simulink model "Ford_T3T6_ArchCnctnDigrm"  (R2016b)
settings: Solver=FixedStepDiscrete  StartTime=0.0  StopTime=10.0  RelTol=1e-3  EnableMultiTasking=on
libraries: canmsglib x15
(part 5 of 15)

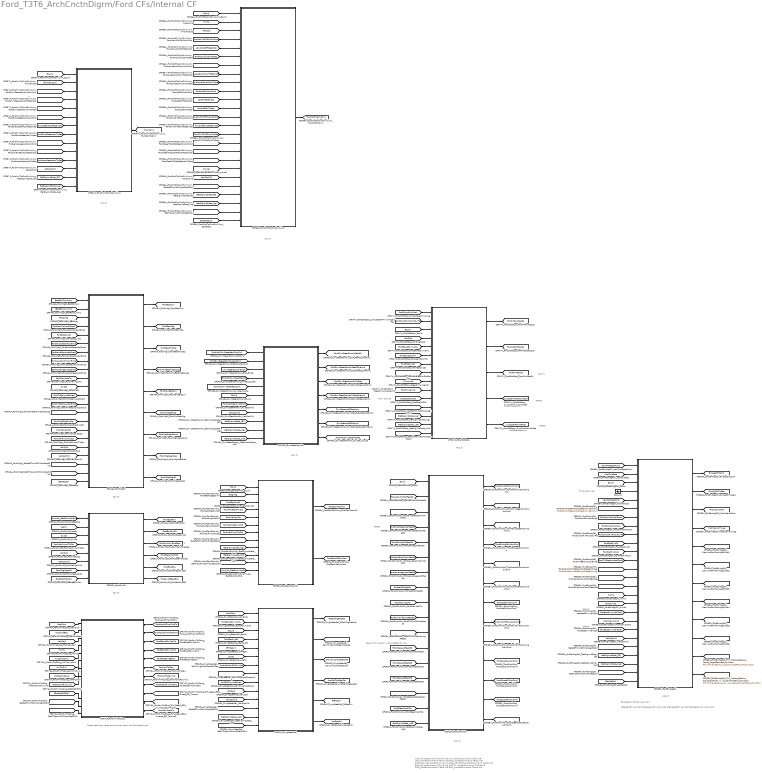
== system Ford_T3T6_ArchCnctnDigrm/Ford CFs/Internal CF ==
  note: CF049
  note: To be removed
  note: A
  note: ??
  note: Takes data from base eps and converts into Ford data type
  note: CAN Tx
  note: SF005
  note: SF005
  note: Spare! Will remain unconnected for now
  note: CF092
  note: LeftLeastDrivenVehicleSpeed
      | kph
      | U-16
      | 1/64
      |
      | RightLeastDrivenVehicleSpeed
      | kph
      | U-16
      | 1/64
  note: EAC_Status
      | Table
      | U-16
      | 1/64
  note: ANC_ArbiterCommand
      | Table
      | U-8
      |
      | LKA_ArbiterCommand
      | Table
      | U-8
      |
      | LDW_ArbiterCommand
      | Table
      | U-8
      |
      | PDC_ArbiterCommand
      | Table
      | U-8
      |
      | PDCLearning_ArbiterCommand
      | Table
      | U-8
      |
      | STDR_ArbiterCommand
      | Table
      | U-8
      |
      | ESA_ArbiterCommand
      | Table
      | U-8
      |
      | LATCTL_ArbiterCommand
      | Table
      | U-8
      |
      | DSR_ArbiterCommand
      | Table
      | U-8
      |
      | EAC_ArbiterCommand
      | Table
      | U-8
  note: ASIL B
  note: ASIL B
  note: ASIL D
  note: ASIL D
  note: ASIL D
  note: ASIL D
  note: ASIL D
  note: StrtStopRateLimit
  note: StrtStopScaleFctr
  note: ASIL D
  note: From DID CF
  note: CF049
  CF046A_FordVltgIf : Subsystem  Tag=1.0.0  Description=This function will inhibit battery voltage diagnostics, define primaryvoltage states and define transitions between battery voltage states
      settings: AttributesFormatString=Version: %<Tag>
  CF047A_FordStrtStop : Subsystem  Tag=1.0.X  Description=Start/Stop is a vehicle event where, to achieve fuel economy,the PCM automatically halts the vehicle engine when the vehicle is stopped and restarts the engine in response to driver commands to resume movement.
      settings: AttributesFormatString=Version: %<Tag>
  CF048A_DrvrSteerRcmdn : Subsystem  Tag=1.0.X  Description=The Driver Steering Recommendation (DSR) function isdesigned to guide the driver to follow/execute a steeringcommand during a split-mu braking or over/understeer condition.This guided steering command is applied in an effort to stabilizethe vehicle and reducing the braking distance in split-mu situations.
      settings: AttributesFormatString=Version: %<Tag>
  CF050A_FordCanDtcInhb : Subsystem  Tag=2.0.X  Description=This function will inhibit requested CAN DTC messagesfor Ford vehicles.This module inhibits CAN DTC messages based on Ford requirements
      settings: AttributesFormatString=Version: %<Tag>
  CF052A_FordSysSt : Subsystem  Tag=1.0.X  Description=Ford System State will handle the internal states and failure modes and output the correct current state to the bus.
      settings: AttributesFormatString=Version: %<Tag>
  CF063A_DrvgSteerSel : Subsystem  Tag=1.0.X  Description=The Driving Steering Select function is a feature which selects different steering modes, safely modifying the steering feel with pre-defined tunings within a given power cycle.
      settings: AttributesFormatString=Version: %<Tag>
  CF065A_FordCmdArbn : Subsystem  Tag=1.0.X  Description=The Ford Arbiter is a function that takes inputs from functions that provide torque overlaysand decides which of those functions may be active and allowed provide a torque overlay
      settings: AttributesFormatString=Version: %<Tag>
  CF066A_FordMotTqCmdOvrlLimr : Subsystem  Tag=1.0.X  Description=The Motor Torque Limiter Function shall sum and limit all output Torque Overlays from Ford features and output them as a value in Motor Nm to be added to the Motor Torque (post-boost curve overlay)
      settings: AttributesFormatString=Version: %<Tag>
  CF067A_FordHwTqCmdOvrlLimr : Subsystem  Tag=1.0.X  Description=The Torque Limiter Function shall sum and limit all inputTorque Overlays from Ford features and output them as avalue in Handwheel Nm to be added to the Handwheel Torque(pre-boost curve overlay)
      settings: AttributesFormatString=Version: %<Tag>
  CF068A_FordExtAgCtrl : Subsystem  Tag=1.0.X  Description=Ford External Angle Control is a function used to process actuationcommands from Ford features into an angle command that can be usedby Nexteer internal functions.
      settings: AttributesFormatString=Version: %<Tag>
  CF076A_FordHwTqCdng : Subsystem  Tag=1.0.X  Description=This function will output various torques in HWNm.It will also calculate an inverse boost curve and outputa percent of available torque for Ford In House Features.
      settings: AttributesFormatString=Version: %<Tag>
  Ground : Ground
  tag scope: DrvrSteerActStPostImc=global, DrvrSteerActStPreImc=global, ExtAgCtrlStsInt=global, ExtAgCtrlTqReq=global, FIH_Read_EPS_Direct_BC_Torque=global, FIH_Read_EPS_Inverse_BC_Torque=global, FIH_Trailer_Backup_Assist_AngleRequest_Function=global, FIH_Trailer_Backup_Assist_External_Angle_ControlStatus_Function=global, FordActvNiblCtrlArbnCmd=global, FordAppldFinalMotTq=global, FordAppldFinalMotTqVld=global, FordBoostCrvAssiTq=global, FordBoostCrvInpTq=global, FordCanDtcInhb=global, FordDrvrSteerRcmdnArbnCmd=global, FordDrvrSteerRcmdnFeatSt=global, FordDrvrSteerRcmdnFeatStPreImc=global, FordDrvrSteerRcmdnTqReq=global, FordDrvrSteerRcmdnTqReqPreImc=global, FordEpsCurr=global, FordEpsEna=global, FordEpsFailr=global, FordEpsLifeCycMod=global, FordEpsSysSt=global, FordEpsVltg=global, FordEvasSteerAssiArbnCmd=global, FordExtAgCtrlArbnCmd=global, FordFeatDircBCTq=global, FordFeatThdSts=global, FordInhbBattVltgDiagc=global, FordInpTqRaw=global, FordInpTqRawVld=global, FordIntPwrReqSt=global, FordIntStrtStopSt=global, FordLaneDprtrWarnArbnCmd=global, FordLaneKeepAssiArbnCmd=global, FordLatCtrlArbnCmd=global, FordMaxAsscTq=global, FordMaxBattCurr=global, FordMinBattVltg=global, FordMotTqCmdOvrl=global, FordPullDriftCmpArbnCmd=global, FordPullDriftCmpLrngArbnCmd=global, FordPwrReqSt=global, FordPwrSplyEnaReq=global, FordReqdFinalMotTq=global, FordSpare1ArbnCmd=global, FordSpare2ArbnCmd=global, FordSpare3ArbnCmd=global, FordSteerDstbcRejctnArbnCmd=global, FordSteerModlSts=global, FordSysStReqEna=global, FordVehDrvrSteerTqReq=global, FordVltgOperRamp=global, FordVltgOperScar=global, FordVltgOperSt=global, HwTqOvrl=global, PosnServoEna=global, PosnServoHwAg=global, RtCalChgReqSts=global, RtReqSrv=global, SelvDrvgModSteerModReq=global, SelvDrvgModSteerSts=global, SemiAutParlParkAgCtrlSts1=global, SemiAutParlParkAgCtrlSts2=global, SemiAutParlParkAgCtrlSts3=global, SemiAutParlParkAgCtrlSts4=global, SemiAutParlParkAgCtrlSts5=global, SemiAutParlParkAgCtrlSts6=global, SysOperMotTqCmdSca=global, SysOperRampRate=global, XcpCalChgReqSts=global, XcpReqSrv=global
  wires:
  [BattRtnCurrAmpr] -> CF046A_FordVltgIf/1(BattRtnCurr)
  [BattRtnCurrImc] -> CF046A_FordVltgIf/2(BattRtnCurrImc)
  [BrdgVltg] -> CF046A_FordVltgIf/3(BattVltg)
  [FordActvParkAssiEnad] -> CF046A_FordVltgIf/4(FordActvParkAssiEnad)
  [FordEpsSysSt] -> CF046A_FordVltgIf/5(FordEpsSysSt)
  [FordEvasSteerAssiEnad] -> CF046A_FordVltgIf/6(FordEvasSteerAssiEnad)
  [FordLaneCentrAssiEnad] -> CF046A_FordVltgIf/7(FordLaneCentrAssiEnad)
  [FordLaneDprtrWarnEnad] -> CF046A_FordVltgIf/8(FordLaneDprtrWarnEnad)
  [FordLaneKeepAssiEnad] -> CF046A_FordVltgIf/9(FordLaneKeepAssiEnad)
  [FordMaxAsscTq] -> CF046A_FordVltgIf/10(FordMaxAsscTq)
  [SysSt] -> CF046A_FordVltgIf/11(FordSysSt)
  [FordTrfcJamAssiEnad] -> CF046A_FordVltgIf/12(FordTrfcJamAssiEnad)
  [FordTrlrBackupAssiEnad] -> CF046A_FordVltgIf/13(FordTrlrBackupAssiEnad)
  [FordVehElecPwrStrtStopSts] -> CF046A_FordVltgIf/14(FordVehElecPwrStrtStopSts)
  [FordVehElecPwrSts] -> CF046A_FordVltgIf/15(FordVehElecPwrSts)
  [FordVehIgnSts] -> CF046A_FordVltgIf/16(FordVehIgnStsQly)
  [FordVehPwrpkTqSts] -> CF046A_FordVltgIf/17(FordVehPwrpkTqSts)
  [VehSpd] -> CF046A_FordVltgIf/18(FordVehSpd)
  [VehSpdVld] -> CF046A_FordVltgIf/19(FordVehSpdVld)
  [GetRefTmr100MicroSec32bit] -> CF046A_FordVltgIf/20(GetRefTmr100MicroSec32bit)
  [GetTiSpan100MicroSec32bit] -> CF046A_FordVltgIf/21(GetTiSpan100MicroSec32bit)
  [SetNtcSts] -> CF046A_FordVltgIf/22(SetNtcSts)
  CF046A_FordVltgIf/1(FordEpsCurr) -> [FordEpsCurr]
  CF046A_FordVltgIf/2(FordEpsVltg) -> [FordEpsVltg]
  CF046A_FordVltgIf/3(FordFeatThdSts) -> [FordFeatThdSts]
  CF046A_FordVltgIf/4(FordInhbBattVltgDiagc) -> [FordInhbBattVltgDiagc]
  CF046A_FordVltgIf/5(FordMaxBattCurr) -> [FordMaxBattCurr]
  CF046A_FordVltgIf/6(FordMinBattVltg) -> [FordMinBattVltg]
  CF046A_FordVltgIf/7(FordVltgOperRamp) -> [FordVltgOperRamp]
  CF046A_FordVltgIf/8(FordVltgOperScar) -> [FordVltgOperScar]
  CF046A_FordVltgIf/9(FordVltgOperSt) -> [FordVltgOperSt]
  [IoHwAb_GetGpioMcuEna] -> CF052A_FordSysSt/1(IoHwAb_GetGpioMcuEna)
  [LoaSt] -> CF052A_FordSysSt/2(LoaSt)
  [SysSt] -> CF052A_FordSysSt/3(SysSt)
  [FordVehPwrpkTqSts] -> CF052A_FordSysSt/4(FordVehPwrpkTqSts)
  [VehSpd] -> CF052A_FordSysSt/5(FordVehSpd)
  [VehSpdVld] -> CF052A_FordSysSt/6(FordVehSpdVld)
  [FordVltgOperSt] -> CF052A_FordSysSt/7(FordVltgOperSt)
  [GetNtcQlfrSts10] -> CF052A_FordSysSt/8(GetNtcQlfrSts)
  CF052A_FordSysSt/1(FordEpsFailr) -> [FordEpsFailr]
  CF052A_FordSysSt/2(FordEpsSysSt) -> [FordEpsSysSt]
  CF052A_FordSysSt/3(FordPwrSplyEnaReq) -> [FordPwrSplyEnaReq]
  CF052A_FordSysSt/4(FordSteerModlSts) -> [FordSteerModlSts]
  [AssiCmd] -> CF076A_FordHwTqCdng/1(AssiCmd)
  [AssiCmdBas] -> CF076A_FordHwTqCdng/2(AssiCmdBas)
  [VehSpd] -> CF076A_FordHwTqCdng/3(FordVehSpd)
  [HwTq] -> CF076A_FordHwTqCdng/4(HwTq)
  [HysCmpCmd] -> CF076A_FordHwTqCdng/5(HwTqHysOvrl)
  [HwTqOvrl] -> CF076A_FordHwTqCdng/6(HwTqOvrl)
  [MotTqCmdSwp] -> CF076A_FordHwTqCdng/7(MotTqCmd)
  [MotTqCmdPwrLimd] -> CF076A_FordHwTqCdng/8(MotTqCmdPwrLimd)
  [GetNtcQlfrSts] -> CF076A_FordHwTqCdng/11(GetNtcQlfrSts)
  [GetRefTmr100MicroSec32bit] -> CF076A_FordHwTqCdng/12(GetRefTmr100MicroSec32bit)
  [GetTiSpan100MicroSec32bit] -> CF076A_FordHwTqCdng/13(GetTiSpan100MicroSec32bit)
  CF076A_FordHwTqCdng/1(FordAppldFinalMotTq) -> [FordAppldFinalMotTq]
  CF076A_FordHwTqCdng/2(FordAppldFinalMotTqVld) -> [FordAppldFinalMotTqVld]
  CF076A_FordHwTqCdng/3(FordBoostCrvAssiTq) -> [FordBoostCrvAssiTq]
  CF076A_FordHwTqCdng/4(FordBoostCrvInpTq) -> [FordBoostCrvInpTq]
  CF076A_FordHwTqCdng/5(FordFeatDircBCTq) -> [FordFeatDircBCTq]
  CF076A_FordHwTqCdng/6(FordInpTqRaw) -> [FordInpTqRaw]
  CF076A_FordHwTqCdng/7(FordInpTqRawVld) -> [FordInpTqRawVld]
  CF076A_FordHwTqCdng/8(FordReqdFinalMotTq) -> [FordReqdFinalMotTq]
  CF076A_FordHwTqCdng/9(FIH_Read_EPS_Direct_BC_Torque) -> [FIH_Read_EPS_Direct_BC_Torque]
  CF076A_FordHwTqCdng/10(FIH_Read_EPS_Inverse_BC_Torque) -> [FIH_Read_EPS_Inverse_BC_Torque]
  [ActvRtIdx] -> CF063A_DrvgSteerSel/1(ActvRtIdx)
  [FordBoostCrvInpTq] -> CF063A_DrvgSteerSel/2(BoostCrvInpTq)
  [EcuId] -> CF063A_DrvgSteerSel/3(EcuId)
  [FordEpsSysSt] -> CF063A_DrvgSteerSel/4(EpsSysSt)
  [FltMtgtn] -> CF063A_DrvgSteerSel/5(FltMtgtn)
  [LoaSt] -> CF063A_DrvgSteerSel/6(LoaSt)
  [FordVehPenSelDrvMod] -> CF063A_DrvgSteerSel/7(SelvDrvgModChassis2Req)
  [FordVehSelDrvModChassisVld] -> CF063A_DrvgSteerSel/8(SelvDrvgModChassisVld)
  [FordSelDrvModEnad] -> CF063A_DrvgSteerSel/9(SelvDrvgModEnad)
  [VehSpd] -> CF063A_DrvgSteerSel/10(VehSpd)
  [VehSpdVld] -> CF063A_DrvgSteerSel/11(VehSpdVld)
  [GetRefTmr100MicroSec32bit] -> CF063A_DrvgSteerSel/12(GetRefTmr100MicroSec32bit)
  [GetSigImcData_u08] -> CF063A_DrvgSteerSel/13(GetSigImcData_u08)
  [GetTiSpan100MicroSec32bit] -> CF063A_DrvgSteerSel/14(GetTiSpan100MicroSec32bit)
  CF063A_DrvgSteerSel/1(RtCalChgReqSts) -> [RtCalChgReqSts]
  CF063A_DrvgSteerSel/2(SelvDrvgModSteerModReq) -> [SelvDrvgModSteerModReq]
  CF063A_DrvgSteerSel/3(SelvDrvgModSteerSts) -> [SelvDrvgModSteerSts]
  CF063A_DrvgSteerSel/4(XcpCalChgReqSts) -> [XcpCalChgReqSts]
  CF063A_DrvgSteerSel/5(RtReqSrv) -> [RtReqSrv]
  CF063A_DrvgSteerSel/6(XcpReqSrv) -> [XcpReqSrv]
  [FordVehDrvrSteerReqCmdVld] -> CF048A_DrvrSteerRcmdn/1(DSRVld)
  [FordDrvrSteerRcmdnArbnCmd] -> CF048A_DrvrSteerRcmdn/2(DSR_ArbiterCmd)
  [DrvrSteerRcmdnEnad] -> CF048A_DrvrSteerRcmdn/3(DSR_Enad)
  [FordVehDrvrSteerReqSts] -> CF048A_DrvrSteerRcmdn/4(DrvSte_D_Stat)
  [FordVehDrvrSteerReqCmd] -> CF048A_DrvrSteerRcmdn/5(DrvSte_Tq_Rq)
  [EcuId] -> CF048A_DrvrSteerRcmdn/6(EcuId)
  [FordVehGearRvsStsVld] -> CF048A_DrvrSteerRcmdn/7(RvsGearVld)
  [VehSpdVld] -> CF048A_DrvrSteerRcmdn/8(VehSpdVld)
  [GetSigImcData_f32] -> CF048A_DrvrSteerRcmdn/9(GetImcSigData_f32)
  [GetSigImcData_logl] -> CF048A_DrvrSteerRcmdn/10(GetImcSigData_logl)
  [GetSigImcData_u08] -> CF048A_DrvrSteerRcmdn/11(GetImcSigData_u08)
  CF048A_DrvrSteerRcmdn/1(DSR_FeatSt_PostImc) -> [FordDrvrSteerRcmdnFeatSt]
  CF048A_DrvrSteerRcmdn/2(DSR_FeatSt_PreImc) -> [FordDrvrSteerRcmdnFeatStPreImc]
  CF048A_DrvrSteerRcmdn/3(DSR_TqReq_PostImc) -> [FordDrvrSteerRcmdnTqReq]
  CF048A_DrvrSteerRcmdn/4(DSR_TqReq_PreImc) -> [FordDrvrSteerRcmdnTqReqPreImc]
  CF048A_DrvrSteerRcmdn/5(DrvSteAct_B_Stat_PostImc) -> [DrvrSteerActStPostImc]
  CF048A_DrvrSteerRcmdn/6(DrvSteAct_B_Stat_PreImc) -> [DrvrSteerActStPreImc]
  CF048A_DrvrSteerRcmdn/7(DrvSte_Tq_Act) -> [FordVehDrvrSteerTqReq]
  [EcuId] -> CF065A_FordCmdArbn/1(EcuId)
  [FordActvNiblCtrlFeatSt] -> CF065A_FordCmdArbn/2(FordActvNiblCtrlFeatSt)
  [FordDrvrSteerRcmdnFeatSt] -> CF065A_FordCmdArbn/3(FordDrvrSteerRcmdnFeatSt)
  [FordEvasSteerAssiFeatSt] -> CF065A_FordCmdArbn/4(FordEvasSteerAssiFeatSt)
  [FordExtAgCtrlFeatSt] -> CF065A_FordCmdArbn/5(FordExtAgCtrlFeatSt)
  [FordLaneDprtrWarnFeatSt] -> CF065A_FordCmdArbn/6(FordLaneDprtrWarnFeatSt)
  [FordLaneKeepAssiFeatSt] -> CF065A_FordCmdArbn/7(FordLaneKeepAssiFeatSt)
  [FordLatCtrlFeatSt] -> CF065A_FordCmdArbn/8(FordLatCtrlFeatSt)
  [FordMaxAsscTq] -> CF065A_FordCmdArbn/9(FordMaxAssiTq)
  [FordPullDriftCmpFeatSt] -> CF065A_FordCmdArbn/10(FordPullDriftCmpFeatSt)
  [FordPullDriftCmpLrngFeatSt] -> CF065A_FordCmdArbn/11(FordPullDriftCmpLrngFeatSt)
  [FordSpare1FeatSt] -> CF065A_FordCmdArbn/12(FordSpare1FeatSt)
  [FordSpare2FeatSt] -> CF065A_FordCmdArbn/13(FordSpare2FeatSt)
  [FordSpare3FeatSt] -> CF065A_FordCmdArbn/14(FordSpare3FeatSt)
  [FordSteerDstbcRejctnFeatSt] -> CF065A_FordCmdArbn/15(FordSteerDstbcRejctnFeatSt)
  [FordSteerModlSts] -> CF065A_FordCmdArbn/16(FordSteerModlSts)
  [GetSigImcData_u08] -> CF065A_FordCmdArbn/17(GetSigImcData_u08)
  CF065A_FordCmdArbn/1(FordActvNiblCtrlArbnCmd) -> [FordActvNiblCtrlArbnCmd]
  CF065A_FordCmdArbn/2(FordDrvrSteerRcmdnArbnCmd) -> [FordDrvrSteerRcmdnArbnCmd]
  CF065A_FordCmdArbn/3(FordEvasSteerAssiArbnCmd) -> [FordEvasSteerAssiArbnCmd]
  CF065A_FordCmdArbn/4(FordExtAgCtrlArbnCmd) -> [FordExtAgCtrlArbnCmd]
  CF065A_FordCmdArbn/5(FordLaneDprtrWarnArbnCmd) -> [FordLaneDprtrWarnArbnCmd]
  CF065A_FordCmdArbn/6(FordLaneKeepAssiArbnCmd) -> [FordLaneKeepAssiArbnCmd]
  CF065A_FordCmdArbn/7(FordLatCtrlArbnCmd) -> [FordLatCtrlArbnCmd]
  CF065A_FordCmdArbn/8(FordPullDriftCmpArbnCmd) -> [FordPullDriftCmpArbnCmd]
  CF065A_FordCmdArbn/9(FordPullDriftCmpLrngArbnCmd) -> [FordPullDriftCmpLrngArbnCmd]
  CF065A_FordCmdArbn/10(FordSpare1ArbnCmd) -> [FordSpare1ArbnCmd]
  CF065A_FordCmdArbn/11(FordSpare2ArbnCmd) -> [FordSpare2ArbnCmd]
  CF065A_FordCmdArbn/12(FordSpare3ArbnCmd) -> [FordSpare3ArbnCmd]
  CF065A_FordCmdArbn/13(FordSteerDstbcRejctnArbnCmd) -> [FordSteerDstbcRejctnArbnCmd]
  [FordCmpdHwPosn] -> CF047A_FordStrtStop/1(CmpdSteerPinionAg)
  [FordCmpdHwPosnQlyFac] -> CF047A_FordStrtStop/2(CmpdSteerPinionAgQlyFac)
  [EcuId] -> CF047A_FordStrtStop/3(EcuId)
  [VehSpd] -> CF047A_FordStrtStop/4(FildVehSpd)
  [FordBoostCrvInpTq] -> CF047A_FordStrtStop/5(FordBoostCrvInpTq)
  [FordCanDtcInhb] -> CF047A_FordStrtStop/6(FordCanDtcInhb)
  [FordEpsSysSt] -> CF047A_FordStrtStop/7(FordEpsSysSt)
  [FordVehElecPwrStrtStopSts] -> CF047A_FordStrtStop/8(FordVehElecPwrStrtStopSts)
  [PinionVel] -> CF047A_FordStrtStop/9(SteerPinionAgVel)
  [FordHwVelVld] -> CF047A_FordStrtStop/10(SteerPinionAgVelVld)
  [StrtStopEnadSt] -> CF047A_FordStrtStop/11(StrtStopDIDSt)
  [GetRefTmr100MicroSec32bit] -> CF047A_FordStrtStop/12(GetRefTmr100MicroSec32bit)
  [GetSigImcData_logl] -> CF047A_FordStrtStop/13(GetSigImcData_logl)
  [GetSigImcData_u08] -> CF047A_FordStrtStop/14(GetSigImcData_u08)
  [GetTiSpan100MicroSec32bit] -> CF047A_FordStrtStop/15(GetTiSpan100MicroSec32bit)
  CF047A_FordStrtStop/1(FordIntPwrReqSt) -> [FordIntPwrReqSt]
  CF047A_FordStrtStop/2(FordIntStrtStopSt) -> [FordIntStrtStopSt]
  CF047A_FordStrtStop/3(FordPwrReqSt) -> [FordPwrReqSt]
  CF047A_FordStrtStop/4(SysOperMotTqCmdSca) -> [SysOperMotTqCmdSca]
  CF047A_FordStrtStop/5(SysOperRampRate) -> [SysOperRampRate]
  [EcuId] -> CF066A_FordMotTqCmdOvrlLimr/1(EcuId)
  [HwTq] -> CF066A_FordMotTqCmdOvrlLimr/2(FildHwTq)
  [VehSpd] -> CF066A_FordMotTqCmdOvrlLimr/3(FildVehSpd)
  [FordActvNiblCtrlArbnCmd] -> CF066A_FordMotTqCmdOvrlLimr/4(FordActvNiblCtrlArbnCmd)
  [ActvNiblCtrlFctCallSts] -> CF066A_FordMotTqCmdOvrlLimr/5(FordActvNiblCtrlFctCallSts)
  [FordActvNiblCtrlTqReq] -> CF066A_FordMotTqCmdOvrlLimr/6(FordActvNiblCtrlTqReq)
  [FordLaneDprtrWarnArbnCmd] -> CF066A_FordMotTqCmdOvrlLimr/7(FordLaneDprtrWarnArbnCmd)
  [LaneDprtrWarnFctCallSts] -> CF066A_FordMotTqCmdOvrlLimr/8(FordLaneDprtrWarnFctCallSts)
  [FordLaneDprtrWarnTqReq] -> CF066A_FordMotTqCmdOvrlLimr/9(FordLaneDprtrWarnTqReq)
  [FordLatCtrlArbnCmd] -> CF066A_FordMotTqCmdOvrlLimr/10(FordLatCtrlArbnCmd)
  [LatCtrlFctCallSts] -> CF066A_FordMotTqCmdOvrlLimr/11(FordLatCtrlFctCallSts)
  [FordLatCtrlTqReq] -> CF066A_FordMotTqCmdOvrlLimr/12(FordLatCtrlTqReq)
  [FordPullDriftCmpArbnCmd] -> CF066A_FordMotTqCmdOvrlLimr/13(FordPullDriftCmpArbnCmd)
  [PullDriftCmpFctCallSts] -> CF066A_FordMotTqCmdOvrlLimr/14(FordPullDriftCmpFctCallSts)
  [FordPullDriftCmpTqReq] -> CF066A_FordMotTqCmdOvrlLimr/15(FordPullDriftCmpTqReq)
  [FordSteerDstbcRejctnArbnCmd] -> CF066A_FordMotTqCmdOvrlLimr/16(FordSteerTqDstbcRejctnArbnCmd)
  [SteerTqDstbcRejctnFctCallSts] -> CF066A_FordMotTqCmdOvrlLimr/17(FordSteerTqDstbcRejctnFctCallSts)
  [FordSteerTqDstbcRejctnTqReq] -> CF066A_FordMotTqCmdOvrlLimr/18(FordSteerTqDstbcRejctnTqReq)
  [HwVel] -> CF066A_FordMotTqCmdOvrlLimr/19(HwVel)
  [VehSpdVld] -> CF066A_FordMotTqCmdOvrlLimr/20(VehSpdVld)
  [GetRefTmr100MicroSec32bit] -> CF066A_FordMotTqCmdOvrlLimr/21(GetRefTmr100MicroSec32bit)
  [GetSigImcData_f32] -> CF066A_FordMotTqCmdOvrlLimr/22(GetSigImcData_f32)
  [GetSigImcData_logl] -> CF066A_FordMotTqCmdOvrlLimr/23(GetSigImcData_logl)
  [GetTiSpan100MicroSec32bit] -> CF066A_FordMotTqCmdOvrlLimr/24(GetTiSpan100MicroSec32bit)
  [SetNtcSts10] -> CF066A_FordMotTqCmdOvrlLimr/25(SetNtcSts)
  CF066A_FordMotTqCmdOvrlLimr/1(FordMotTqOvrl) -> [FordMotTqCmdOvrl]
  [EcuId] -> CF067A_FordHwTqCmdOvrlLimr/1(EcuId)
  [FildVehSpd] -> CF067A_FordHwTqCmdOvrlLimr/2(FildVehSpd)
  [FordDrvrSteerRcmdnArbnCmd] -> CF067A_FordHwTqCmdOvrlLimr/3(FordDrvrSteerRcmdnArbnCmd)
  [FordDrvrSteerRcmdnFctCallSts] -> CF067A_FordHwTqCmdOvrlLimr/4(FordDrvrSteerRcmdnFctCallSts)
  [FordDrvrSteerRcmdnTqReq] -> CF067A_FordHwTqCmdOvrlLimr/5(FordDrvrSteerRcmdnTqReq)
  [FordEvasSteerAssiArbnCmd] -> CF067A_FordHwTqCmdOvrlLimr/6(FordEvasSteerAssiArbnCmd)
  [EvasSteerAssiFctCallSts] -> CF067A_FordHwTqCmdOvrlLimr/7(FordEvasSteerAssiFctCallSts)
  [FordEvasSteerAssiTqReq] -> CF067A_FordHwTqCmdOvrlLimr/8(FordEvasSteerAssiTqReq)
  [FordLaneKeepAssiArbnCmd] -> CF067A_FordHwTqCmdOvrlLimr/9(FordLaneKeepAssiArbnCmd)
  [FordLaneKeepAssiFctCallSts] -> CF067A_FordHwTqCmdOvrlLimr/10(FordLaneKeepAssiFctCallSts)
  [FordLaneKeepAssiTqReq] -> CF067A_FordHwTqCmdOvrlLimr/11(FordLaneKeepAssiTqReq)
  [VehSpdVld] -> CF067A_FordHwTqCmdOvrlLimr/12(VehSpdVld)
  [GetSigImcData_f32] -> CF067A_FordHwTqCmdOvrlLimr/13(GetSigImcData_f32)
  [GetSigImcData_logl] -> CF067A_FordHwTqCmdOvrlLimr/14(GetSigImcData_logl)
  CF067A_FordHwTqCmdOvrlLimr/1(FordColTqOvrl) -> [HwTqOvrl]
  [EcuId] -> CF050A_FordCanDtcInhb/1(EcuId)
  [BrdgVltg] -> CF050A_FordCanDtcInhb/2(FordBattVltgEstimn)
  [FordEpsSysSt] -> CF050A_FordCanDtcInhb/3(FordEpsSysSt)
  [FordVehElecPwrSts] -> CF050A_FordCanDtcInhb/4(FordVehElecPwrSts)
  [FordVehIgnSts] -> CF050A_FordCanDtcInhb/5(FordVehIgnStsQly)
  [FordVehLifeCycMod] -> CF050A_FordCanDtcInhb/6(FordVehLifeCycModQly)
  [FordVehPwrpkTqSts] -> CF050A_FordCanDtcInhb/7(FordVehPwrpkTqSts)
  [GetRefTmr100MicroSec32bit] -> CF050A_FordCanDtcInhb/8(GetRefTmr100MicroSec32bit)
  [GetSigImcData_logl] -> CF050A_FordCanDtcInhb/9(GetSigImcData_logl)
  [GetSigImcData_u08] -> CF050A_FordCanDtcInhb/10(GetSigImcData_u08)
  [GetTiSpan100MicroSec32bit] -> CF050A_FordCanDtcInhb/11(GetTiSpan100MicroSec32bit)
  [IoHwAb_GetGpioMcuEna] -> CF050A_FordCanDtcInhb/12(IoHwAb_GetGpioMcuEna)
  CF050A_FordCanDtcInhb/1(FordCanDtcInhb) -> [FordCanDtcInhb]
  CF050A_FordCanDtcInhb/2(FordEpsLifeCycMod) -> [FordEpsLifeCycMod]
  CF076A_FordHwTqCdng/11(FordMaxAsscTq) -> [FordMaxAsscTq]
  CF052A_FordSysSt/5(FordEpsEna) -> [FordEpsEna]
  CF052A_FordSysSt/6(FordSysStReqEna) -> [FordSysStReqEna]
  [ActvFrntSteerPrsnt] -> CF068A_FordExtAgCtrl/1(ActvFrntSteerPrsnt)
  [AssiCmdBas] -> CF068A_FordExtAgCtrl/2(AssiCmdBas)
  [EcuId] -> CF068A_FordExtAgCtrl/3(EcuId)
  Ground/1 -> CF068A_FordExtAgCtrl/4(ExtAgCtrlDiagcFlg)
  [VehSpdSigCdnd] -> CF068A_FordExtAgCtrl/5(FildVehSpd)
  [FordActvFrntSteerModlSteerWhlAgVldInt] -> CF068A_FordExtAgCtrl/6(FordActvFrntSteerModlSteerWhlAgVldInt)
  [FordActvParkAssiEnad] -> CF068A_FordExtAgCtrl/7(FordActvParkAssiEnad)
  [FordCmpdHwPosn] -> CF068A_FordExtAgCtrl/8(FordCmpdHwPosn)
  [FordCmpdHwPosnQlyFac] -> CF068A_FordExtAgCtrl/9(FordCmpdHwPosnQlyFac)
  [FordEpsSysSt] -> CF068A_FordExtAgCtrl/10(FordEpsSysSt)
  [FordRelHwPosn] -> CF068A_FordExtAgCtrl/11(FordRelHwPosn)
  [FordTrlrBackupAssiEnad] -> CF068A_FordExtAgCtrl/12(FordTrlrBackupAssiEnad)
  [FordVehActvFrntSteerModlSteerWhlAg] -> CF068A_FordExtAgCtrl/13(FordVehActvFrntSteerModlSteerWhlAg)
  [FordVehParkAidModlReqdAgPassd] -> CF068A_FordExtAgCtrl/14(FordVehParkAidModlReqdAg)
  [FordVehParkAidModlReqdStsPassd] -> CF068A_FordExtAgCtrl/15(FordVehParkAidModlReqdSts)
  [HwTq] -> CF068A_FordExtAgCtrl/16(HwTq)
  [FordHwVel] -> CF068A_FordExtAgCtrl/17(HwVel)
  [LeLeastDrvnVehSpd] -> CF068A_FordExtAgCtrl/18(LeLeastDrvnVehSpd)
  [PosnServoCmd] -> CF068A_FordExtAgCtrl/19(PosnServoCmd)
  [RiLeastDrvnVehSpd] -> CF068A_FordExtAgCtrl/20(RiLeastDrvnVehSpd)
  [VehSpdVld] -> CF068A_FordExtAgCtrl/21(VehSpdVld)
  [GetRefTmr100MicroSec32bit] -> CF068A_FordExtAgCtrl/22(GetRefTmr100MicroSec32bit)
  [GetSigImcData_f32] -> CF068A_FordExtAgCtrl/23(GetSigImcData_f32)
  [GetSigImcData_logl] -> CF068A_FordExtAgCtrl/24(GetSigImcData_logl)
  [GetTiSpan100MicroSec32bit] -> CF068A_FordExtAgCtrl/25(GetTiSpan100MicroSec32bit)
  [SetNtcSts] -> CF068A_FordExtAgCtrl/26(SetNtcSts)
  CF068A_FordExtAgCtrl/1(ExtAgCtrlStsInt) -> [ExtAgCtrlStsInt]
  CF068A_FordExtAgCtrl/2(ExtAgCtrlTqReq) -> [ExtAgCtrlTqReq]
  CF068A_FordExtAgCtrl/3(PosnServoEna) -> [PosnServoEna]
  CF068A_FordExtAgCtrl/4(PosnServoHwAg) -> [PosnServoHwAg]
  CF068A_FordExtAgCtrl/5(SemiAutParlParkAgCtrlSts1) -> [SemiAutParlParkAgCtrlSts1]
  CF068A_FordExtAgCtrl/6(SemiAutParlParkAgCtrlSts2) -> [SemiAutParlParkAgCtrlSts2]
  CF068A_FordExtAgCtrl/7(SemiAutParlParkAgCtrlSts3) -> [SemiAutParlParkAgCtrlSts3]
  CF068A_FordExtAgCtrl/8(SemiAutParlParkAgCtrlSts4) -> [SemiAutParlParkAgCtrlSts4]
  CF068A_FordExtAgCtrl/9(SemiAutParlParkAgCtrlSts5) -> [SemiAutParlParkAgCtrlSts5]
  CF068A_FordExtAgCtrl/10(SemiAutParlParkAgCtrlSts6) -> [SemiAutParlParkAgCtrlSts6]
  CF068A_FordExtAgCtrl/11(FIH_Trailer_Backup_Assist_AngleRequest_Function) -> [FIH_Trailer_Backup_Assist_AngleRequest_Function]
  CF068A_FordExtAgCtrl/12(FIH_Trailer_Backup_Assist_External_Angle_ControlStatus_Function) -> [FIH_Trailer_Backup_Assist_External_Angle_ControlStatus_Function]

== system Ford_T3T6_ArchCnctnDigrm/Generate Motor Voltage/CM770A_GtmCfgAndUse ==
  MotCurrEolCalSt : Inport
  SysSt : Inport  Port=2
  MotCtrlMotCurrEolCalSt : Inport  Port=3
  MotCtrlPhaOnTiA : Inport  Port=4
  MotCtrlPhaOnTiB : Inport  Port=5
  MotCtrlPhaOnTiC : Inport  Port=6
  MotCtrlPwmPerd : Inport  Port=7
  IoHwAb_SetFctGpioPhaALowrCmd : Inport  Port=8
  IoHwAb_SetFctGpioPhaAUpprCmd : Inport  Port=9
  IoHwAb_SetFctGpioPhaBLowrCmd : Inport  Port=10
  IoHwAb_SetFctGpioPhaBUpprCmd : Inport  Port=11
  IoHwAb_SetFctGpioPhaCLowrCmd : Inport  Port=12
  IoHwAb_SetFctGpioPhaCUpprCmd : Inport  Port=13
  IoHwAb_SetFctPeriphPhaALowrCmd : Inport  Port=14
  IoHwAb_SetFctPeriphPhaAUpprCmd : Inport  Port=15
  IoHwAb_SetFctPeriphPhaBLowrCmd : Inport  Port=16
  IoHwAb_SetFctPeriphPhaBUpprCmd : Inport  Port=17
  IoHwAb_SetFctPeriphPhaCLowrCmd : Inport  Port=18
  IoHwAb_SetFctPeriphPhaCUpprCmd : Inport  Port=19
  IoHwAb_SetGpioPhaALowrCmd : Inport  Port=20
  IoHwAb_SetGpioPhaAUpprCmd : Inport  Port=21
  IoHwAb_SetGpioPhaBLowrCmd : Inport  Port=22
  IoHwAb_SetGpioPhaBUpprCmd : Inport  Port=23
  IoHwAb_SetGpioPhaCLowrCmd : Inport  Port=24
  IoHwAb_SetGpioPhaCUpprCmd : Inport  Port=25
  PhaOnTiMeasdA : Outport
  PhaOnTiMeasdB : Outport  Port=2
  PhaOnTiMeasdC : Outport  Port=3
  GtmGetSent0Data : Outport  Port=4
  GtmGetSent1Data : Outport  Port=5

== system Ford_T3T6_ArchCnctnDigrm/Generate Motor Voltage/ES300A_SinVltgGenn ==
  MotElecMeclPolarity : Inport
  MotCtrlIvtrFetFltPha : Inport  Port=2
  MotCtrlIvtrFetFltTyp : Inport  Port=3
  MotCtrlMfgEnaSt : Inport  Port=4
  MotCtrlMotAgElec : Inport  Port=5
  MotCtrlMotModlnIdx : Inport  Port=6
  MotCtrlMotPhaAdv : Inport  Port=7
  MotCtrlSwCalEna : Inport  Port=8
  MotCtrlSwCalModlnIdx : Inport  Port=9
  MotCtrlSwCalPosnIdx : Inport  Port=10
  MotCtrlVehSpd : Inport  Port=11
  MotCtrlCmuOffs : Outport
  MotCtrlPhaOnTiA : Outport  Port=2
  MotCtrlPhaOnTiB : Outport  Port=3
  MotCtrlPhaOnTiC : Outport  Port=4
  MotCtrlPhaOnTiSumA : Outport  Port=5
  MotCtrlPhaOnTiSumB : Outport  Port=6
  MotCtrlPhaOnTiSumC : Outport  Port=7
  MotCtrlPwmPerd : Outport  Port=8

== system Ford_T3T6_ArchCnctnDigrm/Generate Steering Command/DF002A_Swp ==
  HwTq : Inport
  MotTqCmd : Inport  Port=2
  VehSpd : Inport  Port=3
  VehSpdVld : Inport  Port=4
  GetRefTmr100MicroSec32bit : Inport  Port=5
  GetTiSpan100MicroSec32bit : Inport  Port=6
  HwTqSwp : Outport
  MotTqCmdSwp : Outport  Port=2

== system Ford_T3T6_ArchCnctnDigrm/Generate Steering Command/Openloop Steering Command ==
  HwTqSwp : Inport
  GenerateSteeringCommand : Subsystem
  System Protection : Subsystem
  MotTqCmd : Outport
  wires:
  HwTqSwp/1 -> GenerateSteeringCommand/1(HwTqSwp)
  GenerateSteeringCommand/1(MotTqCmd) -> MotTqCmd/1
  GenerateSteeringCommand/2(MotTqCmdLimdPreStall) -> System Protection/1(MotTqCmdLimdPreStall)
  System Protection/1(EotAssiSca) -> GenerateSteeringCommand/2(EotAssiSca)
  System Protection/2(EotActvCmd) -> GenerateSteeringCommand/3(EotActvCmd)
  System Protection/3(EotDampgCmd) -> GenerateSteeringCommand/4(EotDampgCmd)
  System Protection/4(EotMotTqLim) -> GenerateSteeringCommand/5(EotMotTqLim)
  System Protection/5(StallMotTqLim) -> GenerateSteeringCommand/6(StallMotTqLim)
  System Protection/6(ThermMotTqLim) -> GenerateSteeringCommand/7(ThermMotTqLim)
  System Protection/7(VehSpdMotTqLim) -> GenerateSteeringCommand/8(VehSpdMotTqLim)

== system Ford_T3T6_ArchCnctnDigrm/Imc Com and Arbn/AR350A_ImcArbn ==
  SetNtcSts : Inport
  GetSigImcDataExtdSts_f32 : Outport
  GetSigImcDataExtdSts_logl : Outport  Port=2
  GetSigImcDataExtdSts_s08 : Outport  Port=3
  GetSigImcDataExtdSts_s16 : Outport  Port=4
  GetSigImcDataExtdSts_s32 : Outport  Port=5
  GetSigImcDataExtdSts_u08 : Outport  Port=6
  GetSigImcDataExtdSts_u16 : Outport  Port=7
  GetSigImcDataExtdSts_u32 : Outport  Port=8
  GetSigImcData_f32 : Outport  Port=9
  GetSigImcData_logl : Outport  Port=10
  GetSigImcData_s08 : Outport  Port=11
  GetSigImcData_s16 : Outport  Port=12
  GetSigImcData_s32 : Outport  Port=13
  GetSigImcData_u08 : Outport  Port=14
  GetSigImcData_u16 : Outport  Port=15
  GetSigImcData_u32 : Outport  Port=16
  GetTxRateGroup : Outport  Port=17
  GetTxSigGroup : Outport  Port=18
  SetRxSigGroup : Outport  Port=19

== system Ford_T3T6_ArchCnctnDigrm/Imc Com and Arbn/CM760A_Uart0CfgAndUse ==
  GetTxRateGroup : Inport
  SetRxSigGroup : Inport  Port=2

== system Ford_T3T6_ArchCnctnDigrm/Imc Com and Arbn/CM765A_Uart1CfgAndUse ==
  GetTxRateGroup : Inport
  SetRxSigGroup : Inport  Port=2

== system Ford_T3T6_ArchCnctnDigrm/Imc Com and Arbn/ES011A_DualEcuIdn ==
  EcuComTiOut : Inport
  GetSigImcData_u08 : Inport  Port=2
  IoHwAb_GetGpioEcuIdnPin1 : Inport  Port=3
  IoHwAb_GetGpioEcuIdnPin2 : Inport  Port=4
  SetNtcSts : Inport  Port=5
  EcuId : Outport  OutMin=0  OutMax=4  OutDataTypeStr=uint8

== system Ford_T3T6_ArchCnctnDigrm/Imc Com and Arbn/SF062B_DualCtrlrOutpMgr ==
  ImcSysSt : Inport
  ImcSysStVld : Inport  Port=2
  MotAndThermProtnLoaMod : Inport  Port=3
  SysSt : Inport  Port=4
  VehSpd : Inport  Port=5
  GetRefTmr100MicroSec32bit : Inport  Port=6
  GetSigImcData_logl : Inport  Port=7
  GetTiSpan100MicroSec32bit : Inport  Port=8
  DualEcuFltMtgtnEna : Outport
  DualEcuFltMtgtnSca : Outport  Port=2
  DualEcuMotCtrlMtgtnEna : Outport  Port=3

== system Ford_T3T6_ArchCnctnDigrm/Imc Com and Arbn/SF063A_ImcSigArbn ==
  EcuIdn : Inport
  HwAg : Inport  Port=2
  HwTq : Inport  Port=3
  MotVelCrf : Inport  Port=4
  PosnServoHwAg : Inport  Port=5
  PosnServoIntgtrSt : Inport  Port=6
  PosnTrakgIntgtrSt1 : Inport  Port=7
  PosnTrakgIntgtrSt2 : Inport  Port=8
  PullCmpLongTermIntgtrSt : Inport  Port=9
  PullCmpShoTermIntgtrSt : Inport  Port=10
  VehSpd : Inport  Port=11
  GetRefTmr100MicroSec32bit : Inport  Port=12
  GetSigImcData_f32 : Inport  Port=13
  GetSigImcData_logl : Inport  Port=14
  GetSigImcData_u08 : Inport  Port=15
  GetTiSpan100MicroSec32bit : Inport  Port=16
  SetNtcSts : Inport  Port=17
  HwAgImcCorrd : Outport
  HwTqImcCorrd : Outport  Port=2
  ImcSysSt : Outport  Port=3
  ImcSysStVld : Outport  Port=4
  MotVelCrfImcCorrd : Outport  Port=5
  PosnServoHwAgImcCorrd : Outport  Port=6
  PosnServoIntgtrOffs : Outport  Port=7
  PosnTrakgArbnFltMtgtnEna : Outport  Port=8
  PosnTrakgIntgtrSt1Offs : Outport  Port=9
  PosnTrakgIntgtrSt2Offs : Outport  Port=10
  PullCmpLongTermIntgtrStOffs : Outport  Port=11
  PullCmpShoTermIntgtrStOffs : Outport  Port=12
  VehSpdImcCorrd : Outport  Port=13

== system Ford_T3T6_ArchCnctnDigrm/Manufacturing/NM002A_CmnMfgSrvIf ==
  MfgEnaSt : Inport
  CmnMfgSrvMaiFct : Inport  Port=2
  ApplTpTxErrIndcn : Outport
  ApplTpRxErrIndcn : Outport  Port=2
  ApplTpRxGetBuf : Outport  Port=3
  ApplTpRxIndcn : Outport  Port=4
  ApplTpTxCfm : Outport  Port=5
  CmnMfgSrvIfImdtTx : Outport  Port=6

== system Ford_T3T6_ArchCnctnDigrm/Manufacturing/NM100A_MotVelCtrl ==
  MotVelCrf : Inport
  GetRefTmr100MicroSec32bit : Inport  Port=2
  GetTiSpan100MicroSec32bit : Inport  Port=3
  SetManTqCmd : Inport  Port=4
  GetCtrlPrm : Outport
  SetCtrlPrm : Outport  Port=2
  StopCtrl : Outport  Port=3
  StrtCtrl : Outport  Port=4

== system Ford_T3T6_ArchCnctnDigrm/Memory/ES006A_NvMProxy ==
  NvM_GetErrorStatus : Inport
  NvM_ReadBlock : Inport  Port=2
  NvM_SetRamBlockStatus : Inport  Port=3
  NvM_WriteBlock : Inport  Port=4
  NvMProxy_ClsChkWr_Oper : Outport
  NvMProxy_GetErrorStatus : Outport  Port=2
  NvMProxy_ReadBlock : Outport  Port=3
  NvMProxy_SetRamBlockStatus : Outport  Port=4
  NvMProxy_WriteBlock : Outport  Port=5
  PortDefinedArgument_GetErrorStatus : Outport  Port=6
  PortDefinedArgument_ReadBlock : Outport  Port=7
  PortDefinedArgument_SetRamBlockStatus : Outport  Port=8
  PortDefinedArgument_WriteBlock : Outport  Port=9

== system Ford_T3T6_ArchCnctnDigrm/Memory/ES400A_TunSelnMngt ==
  DesIninIdx : Inport
  DesRtIdx : Inport  Port=2
  Calc32BitCrc_u32 : Inport  Port=3
  RtCalChgReq : Inport  Port=4
  SetNtcSts : Inport  Port=5
  ActvGroup : Outport
  ActvIninIdx : Outport  Port=2
  ActvRtIdx : Outport  Port=3
  CalCopyCmpl : Outport  Port=4
  CopyCalPageReq : Outport  Port=5
  GetCalPageReq : Outport  Port=6
  GetSegInfoReq : Outport  Port=7
  OnlineTunRamAdrMpg : Outport  Port=8
  SetCalPageReq : Outport  Port=9

== system Ford_T3T6_ArchCnctnDigrm/Memory/SF023A_TunSelnAuthy ==
  HwTq : Inport
  HwVel : Inport  Port=2
  TunSelnRtDi : Inport  Port=3
  VehSpd : Inport  Port=4
  RtCalChgReq : Outport
  XcpCalChgReq : Outport  Port=2

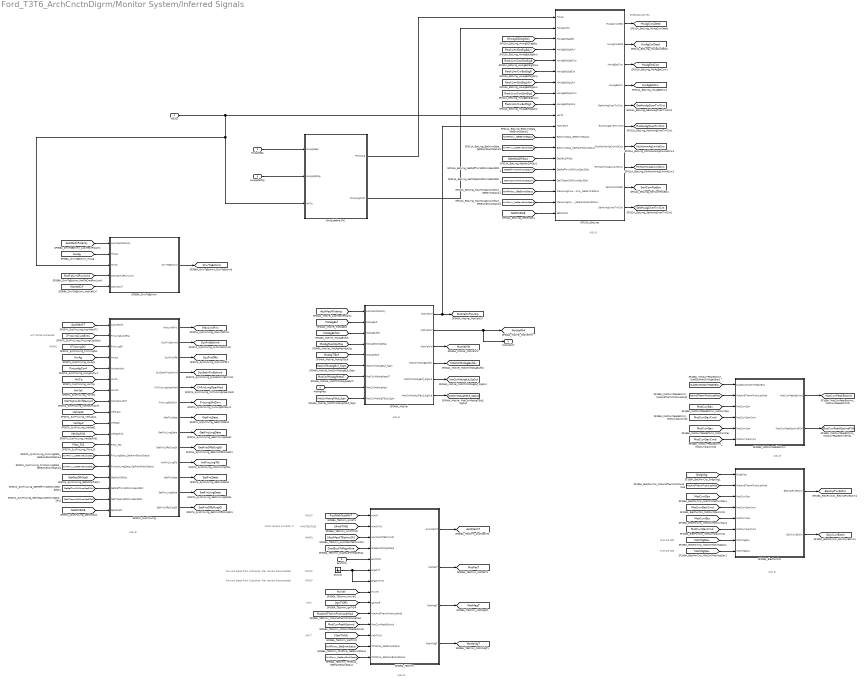
== system Ford_T3T6_ArchCnctnDigrm/Monitor System/Inferred Signals ==
  note: EndStopsLearned
  note: FromAR 300
  note: initial value is currently 0
  note: will not be connected
  note: MM?
  note: MM078/CF100
  note: MM/CF
  note: MM/CF
  note: MM/CF
  note: MM??
  note: ASIL B
  note: ASIL D
  note: ASIL B
  note: ASIL B
  note: ASIL B
  note: ASIL B
  note: No such Signal from Customer. May remain disconnected
  note: No such Signal from Customer. May remain disconnected
  note: FromAR 300
  note: NM001
  note: NM001
  HwTq : Inport
  HwAgMeas : Inport  Port=2
  HwAgIdptSig : Inport  Port=3
  MotAgMecl : Inport  Port=4
  EcuTFild : Inport  Port=5
  Ground : Ground
  HwAg before IMC : Subsystem
  SF006A_TEstimn : Subsystem  Tag=3.1.0  Description=This function provides the estimates of temperature of key motor circuit parameters, namely the power transistor Silicon resistance, motor Copper winding resistance and the motor BEMF coefficient, and if required, for the Assist Mechanism. The temperature estimation is achieved by measuring the controller temperature and using it as an input to a simple lumped parameter system model to estimate the temperatures of the physical parameters which affect the motor circuit parameter values. Additional inputs, namely the Engine and Ambient Temperatures and the Handwheel Velocity, are required to obtain the Assist Mechanism temperature estimate. The design is able to switch between two sets of calibrations based on singl ECU or dual ECU mode of operation.
      settings: AttributesFormatString=Version: %<Tag>
  SF007A_SysFricLrng : Subsystem  Tag=3.2.0  Description="This function improves the steering feel by automatically identifying the EPS gear friction changesfrom the baseline friction and providing the compensation accordingly. The system friction estimationis based on the hysteresis between the total column torque and the hand wheel angle. Due to the factthat the friction from the tire and the road surface is dominating at the low vehicle speed,  and itbecomes less significant as the vehicle speed increases, this function focuses on the friction changes at higher vehicle speeds."
      settings: AttributesFormatString=Version: %<Tag>
  SF011A_EotLrng : Subsystem  Tag=3.2.1  Description="This FDD is focused on using vehicle operational information to learn the appropriate end of travel positions for a given system.  Since the position end stop information is important for such functions as end of travel protection to mechanically protect the gear and since the data can vary from one system to the next, it is important to learn these positions."
      settings: AttributesFormatString=Version: %<Tag>
  SF040A_MotVel : Subsystem  Tag=2.1.1  Description="This function is responsible for computing the rotational velocity of the motor using the motor position signal and the corresponding time-stamp from the motor position function.  A field configurable assist ratio value is provided to scale the motor velocity into handwheel velocity units.  The function consists of two subfunctions, with the Signal Buffering subfunction running at the Motor Control ISR rate, and the Velocity Computation Subfunction running at the same rate as the Assist Functions."
      settings: AttributesFormatString=Version: %<Tag>
  SF056A_DrvrTqEstimn : Subsystem  Tag=1.0.2  Description=This function generates an estimated driver torque using Kalman filter method.
      settings: AttributesFormatString=Version: %<Tag>
  SF108A_MotCurrPeakEstimn : Subsystem  Tag=3.1.0  Description=Motor Current Peak Estimation calculates the peak motor current squared used for thermal duty cycle calculation and temperature estimation.
      settings: AttributesFormatString=Version: %<Tag>
  SF109A_ElecPwrCns : Subsystem  Tag=2.0.0  Description=This function estimates the instantaneous electric power and supply current at the input of the control module for the purpose of transmitting this information over the serial communication bus
      settings: AttributesFormatString=Version: %<Tag>
  MotVelMrf : Outport
  tag scope: AssiMechT=global, ClrFricLrngOperMod=global, DrvrTqEstimd=global, ElecInpPwrEstim=global, FricLrngShtDwn=global, GetFricData=global, GetFricLrngData=global, GetFricOffsOutpDi=global, GetHwAgOverTrvlCnt=global, HwAgCcwDetd=global, HwAgCwDetd=global, HwAgEotCcw=global, HwAgEotCw=global, InitFricLrngTbl=global, MaxLrndFric=global, MotCtrlMotAgBufIdx=global, MotCtrlMotAgBuf_SigOut=global, MotCtrlMotAgTiBuf_SigOut=global, MotCurrPeakEstimd=global, MotCurrPeakEstimdFild=global, MotFetT=global, MotMagT=global, MotVelCrfImcInp=global, MotVelMrf=global, MotVelVld=global, MotWidgT=global, RstHwAgOverTrvlCnt=global, RstMaxHwAgCwAndCcw=global, RtnMaxHwAgCwAndCcw=global, SerlComRstEot=global, SetFricData=global, SetFricLrngData=global, SetFricOffsOutpDi=global, SetHwAgOverTrvlCnt=global, SplyCurrEstim=global, SysFricEstimd=global, SysFricOffs=global, SysSatnFricEstimd=global
  wires:
  [AssiMechPolarity] -> SF056A_DrvrTqEstimn/1(AssiMechPolarity)
  [HwAg] -> SF056A_DrvrTqEstimn/2(HwAg)
  [MotTqCmdPwrLimd] -> SF056A_DrvrTqEstimn/4(MotTqCmdPwrLimd)
  [MotVelCrf] -> SF056A_DrvrTqEstimn/5(MotVelCrf)
  SF056A_DrvrTqEstimn/1(DrvrTqEstimd) -> [DrvrTqEstimd]
  HwAgIdptSig/1 -> HwAg before IMC/2(HwAgIdptSig)
  HwAgMeas/1 -> HwAg before IMC/1(HwAgMeas)
  [AssiMechPolarity] -> SF040A_MotVel/1(AssiMechPolarity)
  [MotAgBuf] -> SF040A_MotVel/2(MotAgBuf)
  [MotAgBufIdx] -> SF040A_MotVel/3(MotAgBufIdx)
  [MotAgMeclIdptSig] -> SF040A_MotVel/4(MotAgMeclIdptSig)
  [MotAgTiBuf] -> SF040A_MotVel/5(MotAgTiBuf)
  [MotCtrlMotAgBuf_SigIn] -> SF040A_MotVel/6(MotCtrlMotAgBuf_SigIn)
  [MotCtrlMotAgMeasTi] -> SF040A_MotVel/7(MotCtrlMotAgMeasTi)
  [MotCtrlMotAgTiBuf_SigIn] -> SF040A_MotVel/9(MotCtrlMotAgTiBuf_SigIn)
  SF040A_MotVel/3(MotVelVld) -> [MotVelVld]
  SF040A_MotVel/4(MotCtrlMotAgBufIdx) -> [MotCtrlMotAgBufIdx]
  SF040A_MotVel/5(MotCtrlMotAgBuf_SigOut) -> [MotCtrlMotAgBuf_SigOut]
  SF040A_MotVel/6(MotCtrlMotAgTiBuf_SigOut) -> [MotCtrlMotAgTiBuf_SigOut]
  SF040A_MotVel/2(MotVelMrf) -> MotVelMrf/1, [MotVelMrf]
  MotAgMecl/1 -> SF040A_MotVel/8(MotCtrlMotAgMecl)
  [BrdgVltg] -> SF109A_ElecPwrCns/1(BrdgVltg)
  [MotAndThermProtnLoaMod] -> SF109A_ElecPwrCns/2(MotAndThermProtnLoaMod)
  [MotCurrDax] -> SF109A_ElecPwrCns/3(MotCurrDax)
  [MotCurrDaxCmd] -> SF109A_ElecPwrCns/4(MotCurrDaxCmd)
  [MotCurrQax] -> SF109A_ElecPwrCns/5(MotCurrQax)
  [MotCurrQaxCmd] -> SF109A_ElecPwrCns/6(MotCurrQaxCmd)
  [MotVltgDax] -> SF109A_ElecPwrCns/7(MotVltgDax)
  [MotVltgQax] -> SF109A_ElecPwrCns/8(MotVltgQax)
  SF109A_ElecPwrCns/1(ElecInpPwrEstim) -> [ElecInpPwrEstim]
  SF109A_ElecPwrCns/2(SplyCurrEstim) -> [SplyCurrEstim]
  [DualEcuMotCtrlMtgtnEna] -> SF108A_MotCurrPeakEstimn/1(DualEcuMotCtrlMtgtnEna)
  [MotAndThermProtnLoaMod] -> SF108A_MotCurrPeakEstimn/2(MotAndThermProtnLoaMod)
  [MotCurrDax] -> SF108A_MotCurrPeakEstimn/3(MotCurrDax)
  [MotCurrDaxCmd] -> SF108A_MotCurrPeakEstimn/4(MotCurrDaxCmd)
  [MotCurrQax] -> SF108A_MotCurrPeakEstimn/5(MotCurrQax)
  [MotCurrQaxCmd] -> SF108A_MotCurrPeakEstimn/6(MotCurrQaxCmd)
  SF108A_MotCurrPeakEstimn/1(MotCurrPeakEstimd) -> [MotCurrPeakEstimd]
  SF108A_MotCurrPeakEstimn/2(MotCurrPeakEstimdFild) -> [MotCurrPeakEstimdFild]
  [FordVehOutdAirT] -> SF006A_TEstimn/1(AmbT)
  [AmbTVld] -> SF006A_TEstimn/2(AmbTVld)
  [AssiMechTEstimnDi] -> SF006A_TEstimn/3(AssiMechTEstimnDi)
  [DualEcuFltMtgtnEna] -> SF006A_TEstimn/4(DualEcuFltMtgtnEna)
  EcuTFild/1 -> SF006A_TEstimn/5(EcuTFild)
  Ground/1 -> SF006A_TEstimn/7(EngOilTVld), SF006A_TEstimn/6(EngOilT)
  [HwVel] -> SF006A_TEstimn/8(HwVel)
  [IgnTiOff] -> SF006A_TEstimn/9(IgnTiOff)
  [MotAndThermProtnLoaMod] -> SF006A_TEstimn/10(MotAndThermProtnLoaMod)
  [MotCurrPeakEstimd] -> SF006A_TEstimn/11(MotCurrPeakEstimd)
  [VehTiVld] -> SF006A_TEstimn/12(VehTiVld)
  [NvMProxy_GetErrorStatus] -> SF006A_TEstimn/13(TFilStVal_GetErrorStatus)
  [NvMProxy_SetRamBlockStatus] -> SF006A_TEstimn/14(TFilStVal_SetRamBlockStatus)
  SF006A_TEstimn/1(AssiMechT) -> [AssiMechT]
  SF006A_TEstimn/2(MotFetT) -> [MotFetT]
  SF006A_TEstimn/3(MotMagT) -> [MotMagT]
  SF006A_TEstimn/4(MotWidgT) -> [MotWidgT]
  [AssiMechT] -> SF007A_SysFricLrng/1(AssiMechT)
  [FricLrngCustEna] -> SF007A_SysFricLrng/2(FricLrngCustEna)
  [FricLrngDi] -> SF007A_SysFricLrng/3(FricLrngDi)
  [HwAg] -> SF007A_SysFricLrng/4(HwAg)
  [PinionAgConf] -> SF007A_SysFricLrng/5(HwAgAuthy)
  [HwTq] -> SF007A_SysFricLrng/6(HwTq)
  [HwVel] -> SF007A_SysFricLrng/7(HwVel)
  [MotTqCmdCrfDampd] -> SF007A_SysFricLrng/8(MotTqCmdCrf)
  [VehLatA] -> SF007A_SysFricLrng/9(VehLatA)
  [VehSpd] -> SF007A_SysFricLrng/10(VehSpd)
  [VehSpdVld] -> SF007A_SysFricLrng/11(VehSpdVld)
  [FltInj_f32] -> SF007A_SysFricLrng/12(FltInj_f32)
  [NvMProxy_SetRamBlockStatus] -> SF007A_SysFricLrng/13(FricLrngData_SetRamBlockStatus)
  [NvMProxy_SetRamBlockStatus] -> SF007A_SysFricLrng/14(FricNonLrngData_SetRamBlockStatus)
  [GetNtcQlfrSts8] -> SF007A_SysFricLrng/15(GetNtcQlfrSts)
  [GetRefTmr100MicroSec32bit] -> SF007A_SysFricLrng/16(GetRefTmr100MicroSec32bit)
  [GetTiSpan100MicroSec32bit] -> SF007A_SysFricLrng/17(GetTiSpan100MicroSec32bit)
  [SetNtcSts8] -> SF007A_SysFricLrng/18(SetNtcSts)
  SF007A_SysFricLrng/1(MaxLrndFric) -> [MaxLrndFric]
  SF007A_SysFricLrng/2(SysFricEstimd) -> [SysFricEstimd]
  SF007A_SysFricLrng/3(SysFricOffs) -> [SysFricOffs]
  SF007A_SysFricLrng/4(SysSatnFricEstimd) -> [SysSatnFricEstimd]
  SF007A_SysFricLrng/5(ClrFricLrngOperMod) -> [ClrFricLrngOperMod]
  SF007A_SysFricLrng/6(FricLrngShtDwn) -> [FricLrngShtDwn]
  SF007A_SysFricLrng/7(GetFricData) -> [GetFricData]
  SF007A_SysFricLrng/8(GetFricLrngData) -> [GetFricLrngData]
  SF007A_SysFricLrng/9(GetFricOffsOutpDi) -> [GetFricOffsOutpDi]
  SF007A_SysFricLrng/10(InitFricLrngTbl) -> [InitFricLrngTbl]
  SF007A_SysFricLrng/11(SetFricData) -> [SetFricData]
  SF007A_SysFricLrng/12(SetFricLrngData) -> [SetFricLrngData]
  SF007A_SysFricLrng/13(SetFricOffsOutpDi) -> [SetFricOffsOutpDi]
  HwAg before IMC/1(PinionAg) -> SF011A_EotLrng/1(HwAg)
  HwAg before IMC/2(PinionAgConf) -> SF011A_EotLrng/2(HwAgAuthy)
  [HwAgDiDiagSts] -> SF011A_EotLrng/3(HwAgDiDiagSts)
  [RackLimrEotSig8Avl] -> SF011A_EotLrng/4(HwAgEotSig0Avl)
  [RackLimrCcwEotSig8] -> SF011A_EotLrng/5(HwAgEotSig0Ccw)
  [RackLimrCwEotSig8] -> SF011A_EotLrng/6(HwAgEotSig0Cw)
  [RackLimrEotSig1Avl] -> SF011A_EotLrng/7(HwAgEotSig1Avl)
  [RackLimrCcwEotSig1] -> SF011A_EotLrng/8(HwAgEotSig1Ccw)
  [RackLimrCwEotSig1] -> SF011A_EotLrng/9(HwAgEotSig1Cw)
  HwTq/1 -> SF011A_EotLrng/10(HwTq), SF056A_DrvrTqEstimn/3(HwTq), HwAg before IMC/3(HwTq)
  SF040A_MotVel/1(MotVelCrf) -> SF011A_EotLrng/11(MotVelCrf), [MotVelCrfImcInp]
  [NvMProxy_GetErrorStatus] -> SF011A_EotLrng/12(EotNvmData_GetErrorStatus)
  [NvMProxy_SetRamBlockStatus] -> SF011A_EotLrng/13(EotNvmData_SetRamBlockStatus)
  [GetNtcQlfrSts] -> SF011A_EotLrng/14(GetNtcQlfrSts)
  [GetRefTmr100MicroSec32bit] -> SF011A_EotLrng/15(GetRefTmr100MicroSec32bit)
  [GetTiSpan100MicroSec32bit] -> SF011A_EotLrng/16(GetTiSpan100MicroSec32bit)
  [NvMProxy_GetErrorStatus] -> SF011A_EotLrng/17(MaxHwAgCwAndCcw_GetErrorStatus)
  [NvMProxy_SetRamBlockStatus] -> SF011A_EotLrng/18(MaxHwAgCwAndCcw_SetRamBlockStatus)
  [SetNtcSts8] -> SF011A_EotLrng/19(SetNtcSts)
  SF011A_EotLrng/1(HwAgCcwDetd) -> [HwAgCcwDetd]
  SF011A_EotLrng/2(HwAgCwDetd) -> [HwAgCwDetd]
  SF011A_EotLrng/3(HwAgEotCcw) -> [HwAgEotCcw]
  SF011A_EotLrng/4(HwAgEotCw) -> [HwAgEotCw]
  SF011A_EotLrng/5(GetHwAgOverTrvlCnt) -> [GetHwAgOverTrvlCnt]
  SF011A_EotLrng/6(RstHwAgOverTrvlCnt) -> [RstHwAgOverTrvlCnt]
  SF011A_EotLrng/7(RstMaxHwAgCwAndCcw) -> [RstMaxHwAgCwAndCcw]
  SF011A_EotLrng/8(RtnMaxHwAgCwAndCcw) -> [RtnMaxHwAgCwAndCcw]
  SF011A_EotLrng/9(SerlComRstEot) -> [SerlComRstEot]
  SF011A_EotLrng/10(SetHwAgOverTrvlCnt) -> [SetHwAgOverTrvlCnt]

== system Ford_T3T6_ArchCnctnDigrm/Monitor System/Measured Signals ==
  MotVelMrf : Inport
  ADC : Subsystem
  BatteryVoltage : Subsystem
  EcuTemp : Subsystem
  HwAg Signal Measurement and  Arbitration : Subsystem
  MotorAngle : Subsystem
  MotorCurrent : Subsystem
  ProcessHandwheelTorqueSignal : Subsystem
  HwTq : Outport
  HwAgMeas : Outport  Port=2
  HwAgIdptSig : Outport  Port=3
  MotAgMech : Outport  Port=4
  EcuTFild : Outport  Port=5
  wires:
  HwAg Signal Measurement and  Arbitration/1(HwAgMeas) -> HwAgMeas/1
  HwAg Signal Measurement and  Arbitration/2(HwAgIdptSig) -> HwAgIdptSig/1
  ProcessHandwheelTorqueSignal/1(HwTq) -> HwTq/1
  MotorAngle/2(MotAgElec) -> MotorCurrent/2(MotAgElec)
  MotorAngle/1(MotAgMecl) -> MotAgMech/1
  MotVelMrf/1 -> MotorCurrent/1(MotVelMrf)
  ADC/1(EcuT) -> EcuTemp/1(EcuT)
  ADC/2(BattVltg) -> BatteryVoltage/1(BattVltg)
  ADC/3(BattVltgSwd1) -> BatteryVoltage/2(BattVltgSwd1)
  EcuTemp/1(EcuTFild) -> EcuTFild/1
